simulink model "motor model"  (R2015b)
settings: Solver=ode23s  StartTime=0.0  StopTime=1  RelTol=1e-3
values from neighbouring files (symbols this model uses):
  Inom = 0.72    [lab.m]
  Ixx = 0.104    [lab.m]
  J = 358*10^(-10)    (= 3.58e-08)    [lab.m]
  Km = 802*10^(-6)    (= 0.000802)    [lab.m]
  Kw = (11900*2*pi/60)^(-1)    (= 0.000802461897942)    [lab.m]
  L = 6*10^(-6)    (= 6e-06)    [lab.m]
  lyambda = (Km*Ixx)/wxx    (= 6.86627353107e-08)    [lab.m]
  Mnom = 499*10^(-6)    (= 0.000499)    [lab.m]
  R = 0.281    [lab.m]
  Unom = 1    [lab.m]
  wnom = 9930*2*pi/60    (= 1039.86716834)    [lab.m]
  wxx = 11600*2*pi/60    (= 1214.74915939)    [lab.m]
settings Model: Creator=semenov2.od  LastModifiedBy=Олег
settings DataIOCC: SaveFormat=Array
settings DebuggingCC: SolverPrmCheckMsg=warning
settings HardwareCC: ProdBitPerPointer=32  ProdLargestAtomicFloat=None  ProdIntDivRoundTo=Undefined  ProdEndianess=Unspecified  ProdWordSize=32  ProdHWDeviceType=32-bit Generic
settings GRTTargetCC: GeneratePreprocessorConditionals=Disable all
settings ConfigComp: CovModelRefEnable=Off  CovSFcnEnable=off

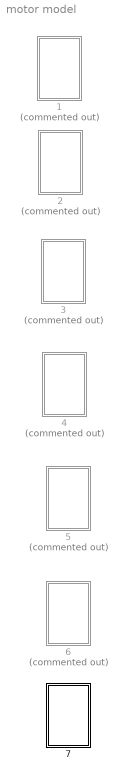
== system motor model ==
  1 : Subsystem  Commented=on
  2 : Subsystem  Commented=on
  3 : Subsystem  Commented=on
  4 : Subsystem  Commented=on
  5 : Subsystem  Commented=on
  6 : Subsystem  Commented=on
  7 : Subsystem

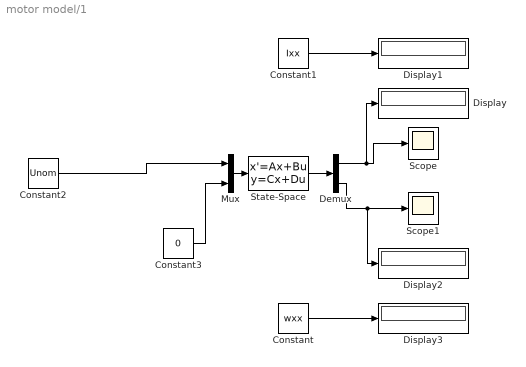
== system motor model/1 ==
  Constant : Constant  Value=wxx
  Constant1 : Constant  Value=Ixx
  Constant2 : Constant  Value=Unom
  Constant3 : Constant  Value=0
  Demux : Demux  Outputs=2
  Display{,1..3} (4 alike) : Display
  Mux : Mux  Inputs=2
  Scope : Scope
  Scope1 : Scope
  State-Space : StateSpace  A=[(-R/L) (-Kw/L);(Km/J) (-lyambda/J)]  B=[(1/L) 0;0 (1/J)]  C=[1 0; 0 1]  D=[0 0; 0 0]  X0=0
  wires:
  Constant3/1 -> Mux/2
  Mux/1 -> State-Space/1
  Constant2/1 -> Mux/1
  Demux/2 -> Display2/1, Scope1/1
  State-Space/1 -> Demux/1
  Demux/1 -> Display/1, Scope/1
  Constant1/1 -> Display1/1
  Constant/1 -> Display3/1

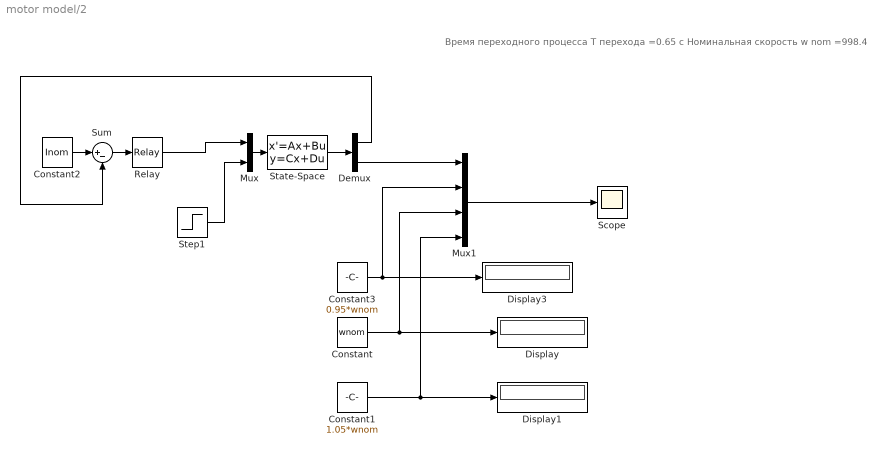
== system motor model/2 ==
  note: Время переходного процесса T перехода =0.65 с
      | Номинальная скорость w nom =998.4
  Constant : Constant  Value=wnom
  Constant1 : Constant  Value=1.05*wnom
  Constant2 : Constant  Value=Inom
  Constant3 : Constant  Value=0.95*wnom
  Demux : Demux  Outputs=2
  Display : Display
  Display1 : Display
  Display3 : Display
  Mux : Mux  Inputs=2
  Mux1 : Mux
  Relay : Relay  OnSwitchValue=Inom/50  OffSwitchValue=-Inom/50  OnOutputValue=Unom  OffOutputValue=-Unom
  Scope : Scope
  State-Space : StateSpace  A=[(-R/L) (-Kw/L);(Km/J) (-lyambda/J)]  B=[(1/L) 0;0 (1/J)]  C=[1 0; 0 1]  D=[0 0; 0 0]  X0=0
  Step1 : Step  Time=0.5  After=-Mnom  SampleTime=0
  Sum : Sum  Inputs=|+-
  wires:
  Constant/1 -> Display/1, Mux1/3
  Step1/1 -> Mux/2
  Demux/1 -> Sum/2
  Constant3/1 -> Display3/1, Mux1/2
  Demux/2 -> Mux1/1
  Constant1/1 -> Display1/1, Mux1/4
  Relay/1 -> Mux/1
  Mux/1 -> State-Space/1
  Mux1/1 -> Scope/1
  State-Space/1 -> Demux/1
  Sum/1 -> Relay/1
  Constant2/1 -> Sum/1

== system motor model/3 ==
  P.3 (б) : Subsystem  Commented=on
  P.3 (в) : Subsystem  Commented=on

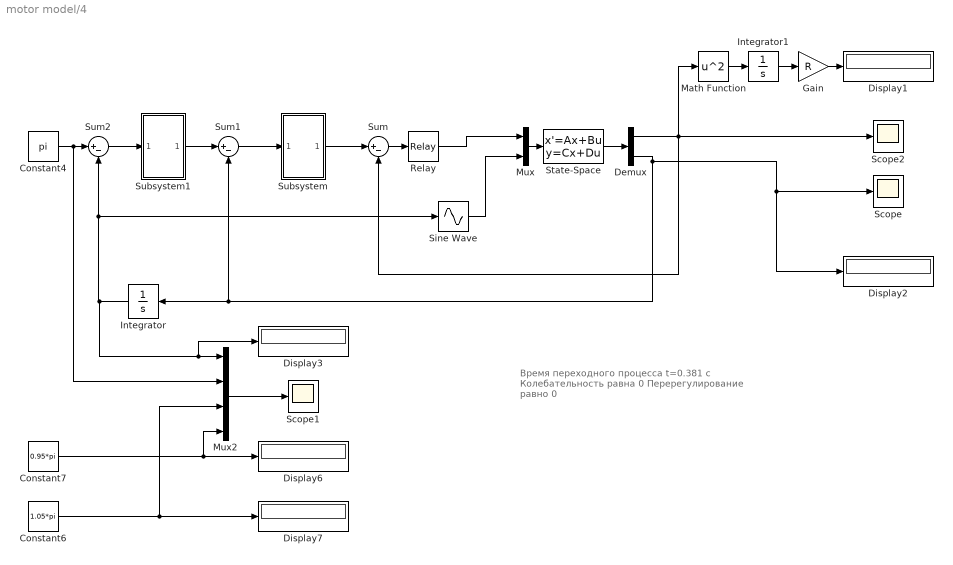
== system motor model/4 ==
  note: Время переходного процесса t=0.381 с
      | Колебательность равна 0
      | Перерегулирование равно 0
  Constant4 : Constant  Value=pi
  Constant6 : Constant  Value=1.05*pi
  Constant7 : Constant  Value=0.95*pi
  Demux : Demux  Outputs=2
  Display{1..3,6..7} (5 alike) : Display
  Gain : Gain  Gain=R
  Integrator : Integrator
  Integrator1 : Integrator
  Math Function : Math  Operator=square  SaturateOnIntegerOverflow=on
  Mux : Mux  Inputs=2
  Mux2 : Mux
  Relay : Relay  OnSwitchValue=Inom/10  OffSwitchValue=-Inom/10  OnOutputValue=Unom  OffOutputValue=-Unom
  Scope : Scope
  Scope1 : Scope
  Scope2 : Scope
  Sine Wave : Sin  TimeSource=Use external signal  Amplitude=-Mnom  SampleTime=0
  State-Space : StateSpace  A=[(-R/L) (-Kw/L);(Km/J) (-lyambda/J)]  B=[(1/L) 0;0 (1/J)]  C=[1 0; 0 1]  D=[0 0; 0 0]  X0=0
  Subsystem : Subsystem
  Subsystem1 : Subsystem
  Sum : Sum  Inputs=|+-
  Sum1 : Sum  Inputs=|+-
  Sum2 : Sum  Inputs=|+-
  wires:
  Constant4/1 -> Mux2/2, Sum2/1
  Constant7/1 -> Display6/1, Mux2/4
  Constant6/1 -> Mux2/3, Display7/1
  Mux2/1 -> Scope1/1
  Sum1/1 -> Subsystem/1(In1)
  Subsystem/1(Out1) -> Sum/1
  Sum/1 -> Relay/1
  State-Space/1 -> Demux/1
  Demux/2 -> Integrator/1, Sum1/2, Scope/1, Display2/1
  Mux/1 -> State-Space/1
  Relay/1 -> Mux/1
  Sine Wave/1 -> Mux/2
  Subsystem1/1(Out1) -> Sum1/1
  Integrator/1 -> Display3/1, Mux2/1, Sine Wave/1, Sum2/2
  Sum2/1 -> Subsystem1/1(In1)
  Demux/1 -> Scope2/1, Math Function/1, Sum/2
  Gain/1 -> Display1/1
  Integrator1/1 -> Gain/1
  Math Function/1 -> Integrator1/1

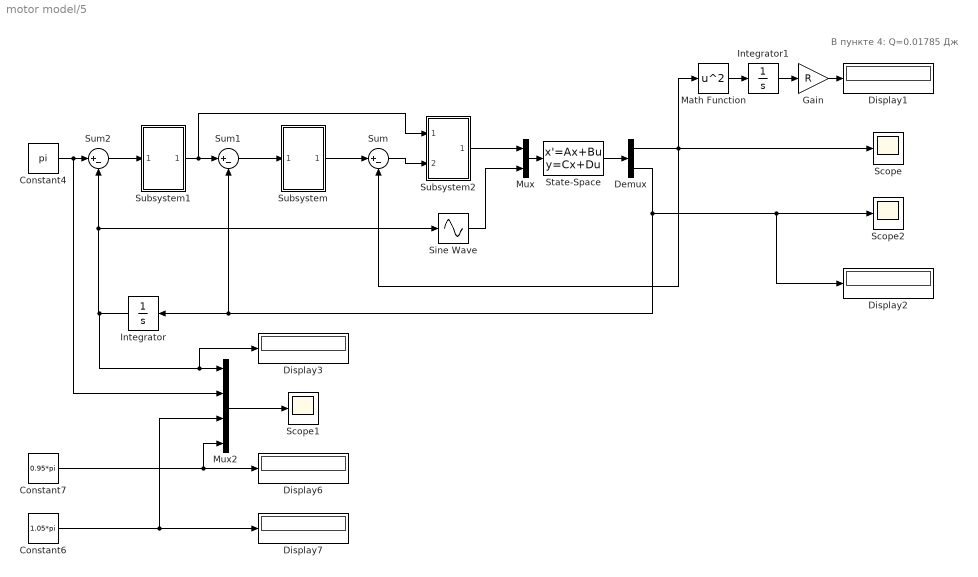
== system motor model/5 ==
  note: В пункте 4: Q=0.01785 Дж
  Constant4 : Constant  Value=pi
  Constant6 : Constant  Value=1.05*pi
  Constant7 : Constant  Value=0.95*pi
  Demux : Demux  Outputs=2
  Display{1..3,6..7} (5 alike) : Display
  Gain : Gain  Gain=R
  Integrator : Integrator
  Integrator1 : Integrator
  Math Function : Math  Operator=square  SaturateOnIntegerOverflow=on
  Mux : Mux  Inputs=2
  Mux2 : Mux
  Scope : Scope
  Scope1 : Scope
  Scope2 : Scope
  Sine Wave : Sin  TimeSource=Use external signal  Amplitude=-Mnom  SampleTime=0
  State-Space : StateSpace  A=[(-R/L) (-Kw/L);(Km/J) (-lyambda/J)]  B=[(1/L) 0;0 (1/J)]  C=[1 0; 0 1]  D=[0 0; 0 0]  X0=0
  Subsystem : Subsystem
  Subsystem1 : Subsystem
  Subsystem2 : Subsystem
  Sum : Sum  Inputs=|+-
  Sum1 : Sum  Inputs=|+-
  Sum2 : Sum  Inputs=|+-
  wires:
  Integrator1/1 -> Gain/1
  Math Function/1 -> Integrator1/1
  Subsystem2/1(Out1) -> Mux/1
  Gain/1 -> Display1/1
  Constant4/1 -> Mux2/2, Sum2/1
  Constant7/1 -> Display6/1, Mux2/4
  Constant6/1 -> Mux2/3, Display7/1
  Mux2/1 -> Scope1/1
  Sum1/1 -> Subsystem/1(In1)
  Subsystem/1(Out1) -> Sum/1
  Sum/1 -> Subsystem2/2(In2)
  State-Space/1 -> Demux/1
  Mux/1 -> State-Space/1
  Demux/1 -> Scope/1, Math Function/1, Sum/2
  Sine Wave/1 -> Mux/2
  Subsystem1/1(Out1) -> Subsystem2/1(In1), Sum1/1
  Integrator/1 -> Display3/1, Mux2/1, Sine Wave/1, Sum2/2
  Sum2/1 -> Subsystem1/1(In1)
  Demux/2 -> Integrator/1, Sum1/2, Display2/1, Scope2/1

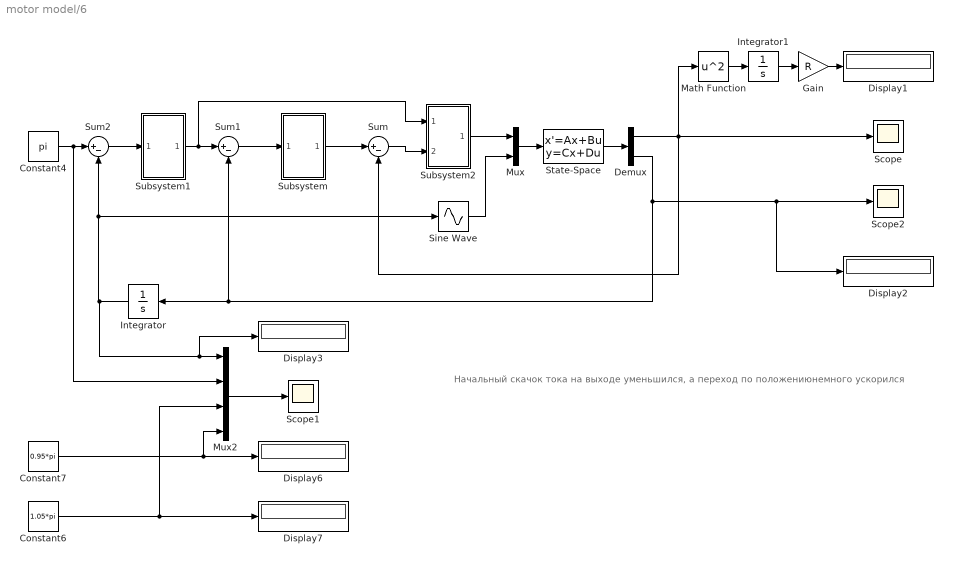
== system motor model/6 ==
  note: Начальный скачок тока на выходе уменьшился, а переход по положениюнемного ускорился
  Constant4 : Constant  Value=pi
  Constant6 : Constant  Value=1.05*pi
  Constant7 : Constant  Value=0.95*pi
  Demux : Demux  Outputs=2
  Display{1..3,6..7} (5 alike) : Display
  Gain : Gain  Gain=R
  Integrator : Integrator
  Integrator1 : Integrator
  Math Function : Math  Operator=square  SaturateOnIntegerOverflow=on
  Mux : Mux  Inputs=2
  Mux2 : Mux
  Scope : Scope
  Scope1 : Scope
  Scope2 : Scope
  Sine Wave : Sin  TimeSource=Use external signal  Amplitude=-Mnom  SampleTime=0
  State-Space : StateSpace  A=[(-R/L) (-Kw/L);(Km/J) (-lyambda/J)]  B=[(1/L) 0;0 (1/J)]  C=[1 0; 0 1]  D=[0 0; 0 0]  X0=0
  Subsystem : Subsystem
  Subsystem1 : Subsystem
  Subsystem2 : Subsystem
  Sum : Sum  Inputs=|+-
  Sum1 : Sum  Inputs=|+-
  Sum2 : Sum  Inputs=|+-
  wires:
  Integrator1/1 -> Gain/1
  Math Function/1 -> Integrator1/1
  Subsystem2/1(Out1) -> Mux/1
  Gain/1 -> Display1/1
  Constant4/1 -> Mux2/2, Sum2/1
  Constant7/1 -> Display6/1, Mux2/4
  Constant6/1 -> Mux2/3, Display7/1
  Mux2/1 -> Scope1/1
  Sum1/1 -> Subsystem/1(In1)
  Subsystem/1(Out1) -> Sum/1
  Sum/1 -> Subsystem2/2(In2)
  State-Space/1 -> Demux/1
  Mux/1 -> State-Space/1
  Demux/1 -> Scope/1, Math Function/1, Sum/2
  Sine Wave/1 -> Mux/2
  Subsystem1/1(Out1) -> Subsystem2/1(In1), Sum1/1
  Integrator/1 -> Display3/1, Mux2/1, Sine Wave/1, Sum2/2
  Sum2/1 -> Subsystem1/1(In1)
  Demux/2 -> Integrator/1, Sum1/2, Display2/1, Scope2/1

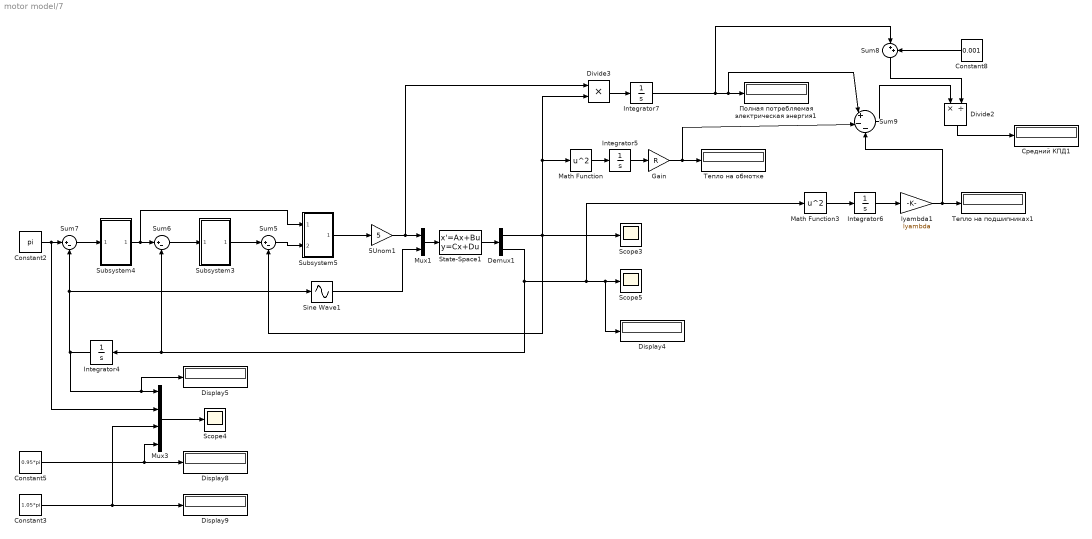
== system motor model/7 ==
  5Unom1 : Gain  Gain=5
  Constant2 : Constant  Value=pi
  Constant3 : Constant  Value=1.05*pi
  Constant5 : Constant  Value=0.95*pi
  Constant8 : Constant  Value=0.001
  Demux1 : Demux  Outputs=2
  Display{4..5,8..9} (4 alike) : Display
  Divide2 : Product  Inputs=*/
  Divide3 : Product  Inputs=**
  Gain : Gain  Gain=R
  Integrator{4..7} (4 alike) : Integrator
  Math Function : Math  Operator=square  SaturateOnIntegerOverflow=on
  Math Function3 : Math  Operator=square  SaturateOnIntegerOverflow=on
  Mux1 : Mux  Inputs=2
  Mux3 : Mux
  Scope3 : Scope
  Scope4 : Scope
  Scope5 : Scope
  Sine Wave1 : Sin  TimeSource=Use external signal  Amplitude=-Mnom  SampleTime=0
  State-Space1 : StateSpace  A=[(-R/L) (-Kw/L);(Km/J) (-lyambda/J)]  B=[(1/L) 0;0 (1/J)]  C=[1 0; 0 1]  D=[0 0; 0 0]  X0=0
  Subsystem3 : Subsystem
  Subsystem4 : Subsystem
  Subsystem5 : Subsystem
  Sum5 : Sum  Inputs=|+-
  Sum6 : Sum  Inputs=|+-
  Sum7 : Sum  Inputs=|+-
  Sum8 : Sum  Inputs=|++
  Sum9 : Sum  Inputs=|+|-|-
  lyambda1 : Gain  Gain=lyambda
  Полная потребляемая электрическая энергия1 : Display
  Средний КПД1 : Display
  Тепло на обмотке : Display
  Тепло на подшипниках1 : Display
  wires:
  Integrator5/1 -> Gain/1
  Math Function/1 -> Integrator5/1
  Constant2/1 -> Mux3/2, Sum7/1
  Constant5/1 -> Display8/1, Mux3/4
  Constant3/1 -> Mux3/3, Display9/1
  Mux3/1 -> Scope4/1
  Sum6/1 -> Subsystem3/1(In1)
  Subsystem3/1(Out1) -> Sum5/1
  Sum5/1 -> Subsystem5/2(In2)
  State-Space1/1 -> Demux1/1
  Demux1/1 -> Scope3/1, Divide3/2, Math Function/1, Sum5/2
  Sine Wave1/1 -> Mux1/2
  Subsystem4/1(Out1) -> Subsystem5/1(In1), Sum6/1
  Integrator4/1 -> Display5/1, Mux3/1, Sine Wave1/1, Sum7/2
  Sum7/1 -> Subsystem4/1(In1)
  Demux1/2 -> Math Function3/1, Display4/1, Scope5/1, Integrator4/1, Sum6/2
  Mux1/1 -> State-Space1/1
  Subsystem5/1(Out1) -> 5Unom1/1
  Constant8/1 -> Sum8/2
  Sum9/1 -> Divide2/1
  Integrator6/1 -> lyambda1/1
  Gain/1 -> Тепло на обмотке/1, Sum9/2
  Math Function3/1 -> Integrator6/1
  lyambda1/1 -> Sum9/3, Тепло на подшипниках1/1
  Divide2/1 -> Средний КПД1/1
  Sum8/1 -> Divide2/2
  Divide3/1 -> Integrator7/1
  Integrator7/1 -> Sum8/1, Sum9/1, Полная потребляемая электрическая энергия1/1
  5Unom1/1 -> Divide3/1, Mux1/1

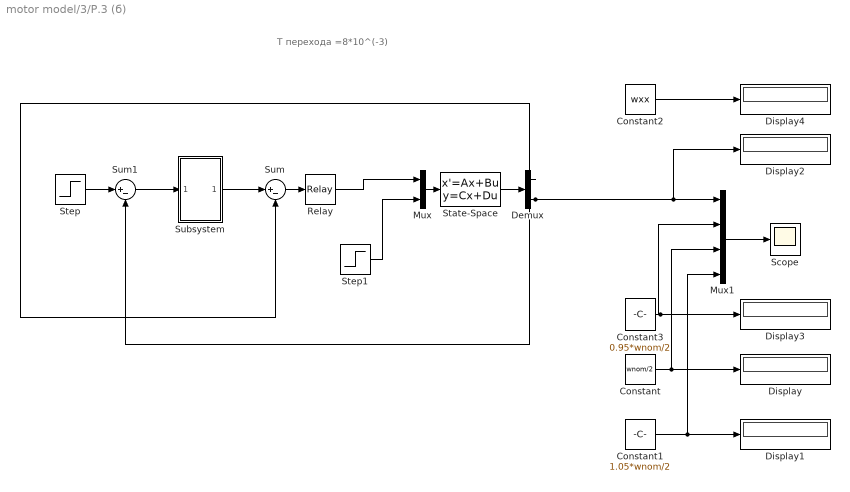
== system motor model/3/P.3 (б) ==
  note: Т перехода =8*10^(-3)
  Constant : Constant  Value=wnom/2
  Constant1 : Constant  Value=1.05*wnom/2
  Constant2 : Constant  Value=wxx
  Constant3 : Constant  Value=0.95*wnom/2
  Demux : Demux  Outputs=2
  Display{,1..4} (5 alike) : Display
  Mux : Mux  Inputs=2
  Mux1 : Mux
  Relay : Relay  OnSwitchValue=Inom/10  OffSwitchValue=-Inom/10  OnOutputValue=Unom  OffOutputValue=-Unom  ZeroCross=off
  Scope : Scope
  State-Space : StateSpace  A=[(-R/L) (-Kw/L);(Km/J) (-lyambda/J)]  B=[(1/L) 0;0 (1/J)]  C=[1 0; 0 1]  D=[0 0; 0 0]  X0=0
  Step : Step  Time=0  After=wnom/2  SampleTime=0
  Step1 : Step  Time=0.5  After=-Mnom  SampleTime=0
  Subsystem : Subsystem
  Sum : Sum  Inputs=|+-
  Sum1 : Sum  Inputs=|+-
  wires:
  Step/1 -> Sum1/1
  Constant/1 -> Display/1, Mux1/3
  Step1/1 -> Mux/2
  Demux/1 -> Sum/2
  Constant3/1 -> Mux1/2, Display3/1
  Demux/2 -> Sum1/2, Display2/1, Mux1/1
  Constant1/1 -> Display1/1, Mux1/4
  Relay/1 -> Mux/1
  Mux/1 -> State-Space/1
  Mux1/1 -> Scope/1
  State-Space/1 -> Demux/1
  Sum/1 -> Relay/1
  Subsystem/1(Out1) -> Sum/1
  Sum1/1 -> Subsystem/1(In1)
  Constant2/1 -> Display4/1

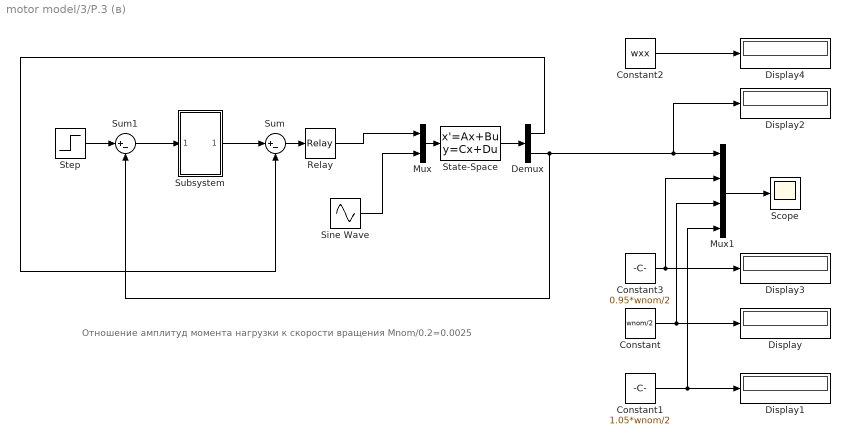
== system motor model/3/P.3 (в) ==
  note: Отношение амплитуд момента нагрузки к скорости вращения
      | Mnom/0.2=0.0025
  Constant : Constant  Value=wnom/2
  Constant1 : Constant  Value=1.05*wnom/2
  Constant2 : Constant  Value=wxx
  Constant3 : Constant  Value=0.95*wnom/2
  Demux : Demux  Outputs=2
  Display{,1..4} (5 alike) : Display
  Mux : Mux  Inputs=2
  Mux1 : Mux
  Relay : Relay  OnSwitchValue=Inom/10  OffSwitchValue=-Inom/10  OnOutputValue=Unom  OffOutputValue=-Unom  ZeroCross=off
  Scope : Scope
  Sine Wave : Sin  Amplitude=-Mnom  Frequency=wnom/1000  SampleTime=0
  State-Space : StateSpace  A=[(-R/L) (-Kw/L);(Km/J) (-lyambda/J)]  B=[(1/L) 0;0 (1/J)]  C=[1 0; 0 1]  D=[0 0; 0 0]  X0=0
  Step : Step  Time=0  After=wnom/2  SampleTime=0
  Subsystem : Subsystem
  Sum : Sum  Inputs=|+-
  Sum1 : Sum  Inputs=|+-
  wires:
  Constant2/1 -> Display4/1
  Sum1/1 -> Subsystem/1(In1)
  Subsystem/1(Out1) -> Sum/1
  Sum/1 -> Relay/1
  State-Space/1 -> Demux/1
  Mux1/1 -> Scope/1
  Mux/1 -> State-Space/1
  Relay/1 -> Mux/1
  Constant1/1 -> Display1/1, Mux1/4
  Demux/2 -> Sum1/2, Display2/1, Mux1/1
  Constant3/1 -> Mux1/2, Display3/1
  Demux/1 -> Sum/2
  Sine Wave/1 -> Mux/2
  Constant/1 -> Display/1, Mux1/3
  Step/1 -> Sum1/1

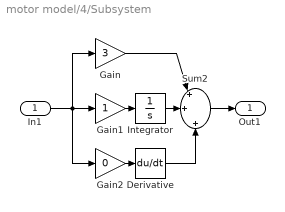
== system motor model/4/Subsystem ==
  In1 : Inport
  Derivative : Derivative
  Gain : Gain  Gain=3
  Gain1 : Gain
  Gain2 : Gain  Gain=0
  Integrator : Integrator
  Sum2 : Sum  Inputs=|+|+||+
  Out1 : Outport
  wires:
  Gain/1 -> Sum2/1
  In1/1 -> Gain2/1, Gain1/1, Gain/1
  Sum2/1 -> Out1/1
  Integrator/1 -> Sum2/2
  Derivative/1 -> Sum2/3
  Gain1/1 -> Integrator/1
  Gain2/1 -> Derivative/1

== system motor model/4/Subsystem1 ==
  In1 : Inport
  Derivative : Derivative
  Gain : Gain  Gain=8
  Gain1 : Gain  Gain=0
  Gain2 : Gain  Gain=0
  Integrator : Integrator
  Sum2 : Sum  Inputs=|+|+||+
  Out1 : Outport
  wires:
  Gain/1 -> Sum2/1
  In1/1 -> Gain2/1, Gain1/1, Gain/1
  Sum2/1 -> Out1/1
  Integrator/1 -> Sum2/2
  Derivative/1 -> Sum2/3
  Gain1/1 -> Integrator/1
  Gain2/1 -> Derivative/1

== system motor model/5/Subsystem ==
  In1 : Inport
  Derivative : Derivative
  Gain : Gain  Gain=3
  Gain1 : Gain
  Gain2 : Gain  Gain=0
  Integrator : Integrator
  Sum2 : Sum  Inputs=|+|+||+
  Out1 : Outport
  wires:
  Gain/1 -> Sum2/1
  In1/1 -> Gain2/1, Gain1/1, Gain/1
  Sum2/1 -> Out1/1
  Integrator/1 -> Sum2/2
  Derivative/1 -> Sum2/3
  Gain1/1 -> Integrator/1
  Gain2/1 -> Derivative/1

== system motor model/5/Subsystem1 ==
  In1 : Inport
  Derivative : Derivative
  Gain : Gain  Gain=8
  Gain1 : Gain  Gain=0
  Gain2 : Gain  Gain=0
  Integrator : Integrator
  Sum2 : Sum  Inputs=|+|+||+
  Out1 : Outport
  wires:
  Gain/1 -> Sum2/1
  In1/1 -> Gain2/1, Gain1/1, Gain/1
  Sum2/1 -> Out1/1
  Integrator/1 -> Sum2/2
  Derivative/1 -> Sum2/3
  Gain1/1 -> Integrator/1
  Gain2/1 -> Derivative/1

== system motor model/5/Subsystem2 ==
  In1 : Inport
  In2 : Inport  Port=2
  Relay : Relay  OnSwitchValue=Inom/10  OffSwitchValue=-Inom/10  OnOutputValue=Unom
  Relay1 : Relay  OnSwitchValue=Inom/10  OffSwitchValue=-Inom/10  OnOutputValue=0  OffOutputValue=-Unom
  Switch : Switch  Criteria=u2 > Threshold
  Out1 : Outport
  wires:
  In2/1 -> Relay1/1, Relay/1
  In1/1 -> Switch/2
  Switch/1 -> Out1/1
  Relay1/1 -> Switch/3
  Relay/1 -> Switch/1

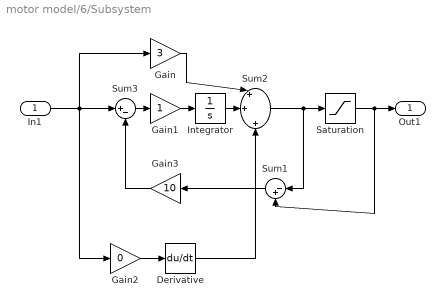
== system motor model/6/Subsystem ==
  In1 : Inport
  Derivative : Derivative
  Gain : Gain  Gain=3
  Gain1 : Gain
  Gain2 : Gain  Gain=0
  Gain3 : Gain  Gain=10
  Integrator : Integrator
  Saturation : Saturate  UpperLimit=Inom  LowerLimit=-Inom
  Sum1 : Sum  Inputs=|-+
  Sum2 : Sum  Inputs=|+|+||+
  Sum3 : Sum  Inputs=|+-
  Out1 : Outport
  wires:
  Gain/1 -> Sum2/1
  In1/1 -> Sum3/1, Gain/1, Gain2/1
  Integrator/1 -> Sum2/2
  Derivative/1 -> Sum2/3
  Gain1/1 -> Integrator/1
  Gain2/1 -> Derivative/1
  Sum2/1 -> Sum1/1, Saturation/1
  Saturation/1 -> Out1/1, Sum1/2
  Sum1/1 -> Gain3/1
  Sum3/1 -> Gain1/1
  Gain3/1 -> Sum3/2

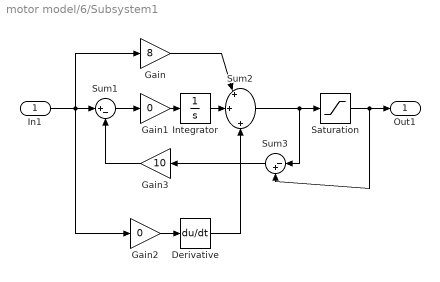
== system motor model/6/Subsystem1 ==
  In1 : Inport
  Derivative : Derivative
  Gain : Gain  Gain=8
  Gain1 : Gain  Gain=0
  Gain2 : Gain  Gain=0
  Gain3 : Gain  Gain=10
  Integrator : Integrator
  Saturation : Saturate  UpperLimit=wnom  LowerLimit=-wnom
  Sum1 : Sum  Inputs=|+-
  Sum2 : Sum  Inputs=|+|+||+
  Sum3 : Sum  Inputs=|-+
  Out1 : Outport
  wires:
  Gain/1 -> Sum2/1
  In1/1 -> Sum1/1, Gain2/1, Gain/1
  Integrator/1 -> Sum2/2
  Derivative/1 -> Sum2/3
  Gain1/1 -> Integrator/1
  Gain2/1 -> Derivative/1
  Sum1/1 -> Gain1/1
  Sum2/1 -> Sum3/1, Saturation/1
  Saturation/1 -> Sum3/2, Out1/1
  Sum3/1 -> Gain3/1
  Gain3/1 -> Sum1/2

== system motor model/6/Subsystem2 ==
  In1 : Inport
  In2 : Inport  Port=2
  Relay : Relay  OnSwitchValue=Inom/10  OffSwitchValue=-Inom/10  OnOutputValue=Unom
  Relay1 : Relay  OnSwitchValue=Inom/10  OffSwitchValue=-Inom/10  OnOutputValue=0  OffOutputValue=-Unom
  Switch : Switch  Criteria=u2 > Threshold
  Out1 : Outport
  wires:
  In2/1 -> Relay1/1, Relay/1
  In1/1 -> Switch/2
  Switch/1 -> Out1/1
  Relay1/1 -> Switch/3
  Relay/1 -> Switch/1

== system motor model/7/Subsystem3 ==
  In1 : Inport
  Derivative : Derivative
  Gain : Gain  Gain=3
  Gain1 : Gain
  Gain2 : Gain  Gain=0
  Integrator : Integrator
  Sum2 : Sum  Inputs=|+|+||+
  Out1 : Outport
  wires:
  Gain/1 -> Sum2/1
  In1/1 -> Gain2/1, Gain1/1, Gain/1
  Sum2/1 -> Out1/1
  Integrator/1 -> Sum2/2
  Derivative/1 -> Sum2/3
  Gain1/1 -> Integrator/1
  Gain2/1 -> Derivative/1

== system motor model/7/Subsystem4 ==
  In1 : Inport
  Derivative : Derivative
  Gain : Gain  Gain=8
  Gain1 : Gain  Gain=0
  Gain2 : Gain  Gain=0
  Integrator : Integrator
  Sum2 : Sum  Inputs=|+|+||+
  Out1 : Outport
  wires:
  Gain/1 -> Sum2/1
  In1/1 -> Gain2/1, Gain1/1, Gain/1
  Sum2/1 -> Out1/1
  Integrator/1 -> Sum2/2
  Derivative/1 -> Sum2/3
  Gain1/1 -> Integrator/1
  Gain2/1 -> Derivative/1

== system motor model/7/Subsystem5 ==
  In1 : Inport
  In2 : Inport  Port=2
  Relay : Relay  OnSwitchValue=Inom/10  OffSwitchValue=-Inom/10  OnOutputValue=Unom
  Relay1 : Relay  OnSwitchValue=Inom/10  OffSwitchValue=-Inom/10  OnOutputValue=0  OffOutputValue=-Unom
  Switch : Switch  Criteria=u2 > Threshold
  Out1 : Outport
  wires:
  In2/1 -> Relay1/1, Relay/1
  In1/1 -> Switch/2
  Switch/1 -> Out1/1
  Relay1/1 -> Switch/3
  Relay/1 -> Switch/1

== system motor model/3/P.3 (б)/Subsystem ==
  In1 : Inport
  Derivative : Derivative
  Gain : Gain  Gain=3
  Gain1 : Gain
  Gain2 : Gain  Gain=0
  Integrator : Integrator  InitialCondition=1
  Sum2 : Sum  Inputs=|+|+||+
  Out1 : Outport
  wires:
  Gain/1 -> Sum2/1
  In1/1 -> Gain2/1, Gain1/1, Gain/1
  Sum2/1 -> Out1/1
  Integrator/1 -> Sum2/2
  Derivative/1 -> Sum2/3
  Gain1/1 -> Integrator/1
  Gain2/1 -> Derivative/1

== system motor model/3/P.3 (в)/Subsystem ==
  In1 : Inport
  Derivative : Derivative
  Gain : Gain  Gain=3
  Gain1 : Gain
  Gain2 : Gain  Gain=0
  Integrator : Integrator
  Sum2 : Sum  Inputs=|+|+||+
  Out1 : Outport
  wires:
  Gain/1 -> Sum2/1
  In1/1 -> Gain2/1, Gain1/1, Gain/1
  Sum2/1 -> Out1/1
  Integrator/1 -> Sum2/2
  Derivative/1 -> Sum2/3
  Gain1/1 -> Integrator/1
  Gain2/1 -> Derivative/1
